simulink model "TASK4"  (R2019a)
settings: Solver=VariableStepAuto  StartTime=0.0  StopTime=30  RelTol=1e-3
values from neighbouring files (symbols this model uses):
  A = [0,mf*g*h/Jconst,0,-(mf*g)/Jconst;1,0,0,0;0,-g,0,0;0,0,1,0]    [Dharmesh_DCS_LAB_Script.m]
  B = [1/Jconst;0;0;0]    [Dharmesh_DCS_LAB_Script.m]
  C = eye(4)    [Dharmesh_DCS_LAB_Script.m]
  D = [0;0;0;0]    [Dharmesh_DCS_LAB_Script.m]
  g = 9.81    [Dharmesh_DCS_LAB_Script.m]
  h = 0.1    [Dharmesh_DCS_LAB_Script.m]
  Jconst = Jb+mf*h^2    (= 0.501)    [Dharmesh_DCS_LAB_Script.m]
  K = q * (alpha(5)*eye(4) + alpha(4)*A + alpha(3)*A^2 + alpha(2)*A^3 + A^4)    [Dharmesh_DCS_LAB_Script.m]
  mf = 0.1    [Dharmesh_DCS_LAB_Script.m]
  P = 1/(Ct*inv((B*K)-A)*B)    [Dharmesh_DCS_LAB_Script.m]
settings Model: Creator=Admin  LastModifiedBy=Admin

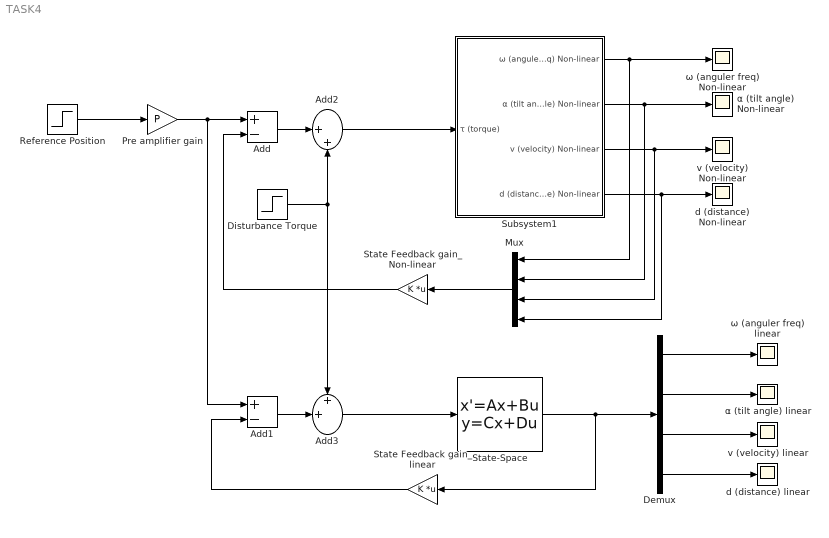
== system TASK4 ==
  "      ω (anguler freq) Non-linear" : Scope
  Add : Sum  Inputs=+-
  Add1 : Sum  Inputs=+-
  Add2 : Sum  Inputs=|++
  Add3 : Sum  Inputs=++|
  Demux : Demux
  Disturbance Torque : Step  Time=15  After=0.1  SampleTime=0
  Mux : Mux
  Pre amplifier gain : Gain  Gain=P
  Reference Position : Step  Time=0  SampleTime=0
  State Feedback gain_Non-linear : Gain  Gain=K  Multiplication=Matrix(K*u) (u vector)
  State Feedback gain_linear : Gain  Gain=K  Multiplication=Matrix(K*u) (u vector)
  State-Space : StateSpace  A=A  B=B  C=C  D=D  InitialCondition=0
  Subsystem1 : Subsystem
  d (distance) Non-linear : Scope
  d (distance) linear : Scope
  v (velocity) Non-linear : Scope
  v (velocity) linear : Scope
  α (tilt angle) Non-linear : Scope
  α (tilt angle) linear : Scope
  ω (anguler freq) linear : Scope
  wires:
  State Feedback gain_Non-linear/1 -> Add/2
  Reference Position/1 -> Pre amplifier gain/1
  State Feedback gain_linear/1 -> Add1/2
  Pre amplifier gain/1 -> Add/1, Add1/1
  Mux/1 -> State Feedback gain_Non-linear/1
  State-Space/1 -> State Feedback gain_linear/1, Demux/1
  Demux/1 -> ω (anguler freq) linear/1
  Demux/2 -> α (tilt angle) linear/1
  Demux/4 -> d (distance) linear/1
  Demux/3 -> v (velocity) linear/1
  Subsystem1/4(d (distance) Non-linear) -> Mux/4, d (distance) Non-linear/1
  Subsystem1/3(v (velocity) Non-linear) -> Mux/3, v (velocity) Non-linear/1
  Subsystem1/2(α (tilt angle) Non-linear) -> Mux/2, α (tilt angle) Non-linear/1
  Subsystem1/1(ω (anguler freq) Non-linear) -> Mux/1, "      ω (anguler freq) Non-linear"/1
  Add2/1 -> Subsystem1/1(τ (torque))
  Add/1 -> Add2/1
  Add1/1 -> Add3/2
  Add3/1 -> State-Space/1
  Disturbance Torque/1 -> Add2/2, Add3/1

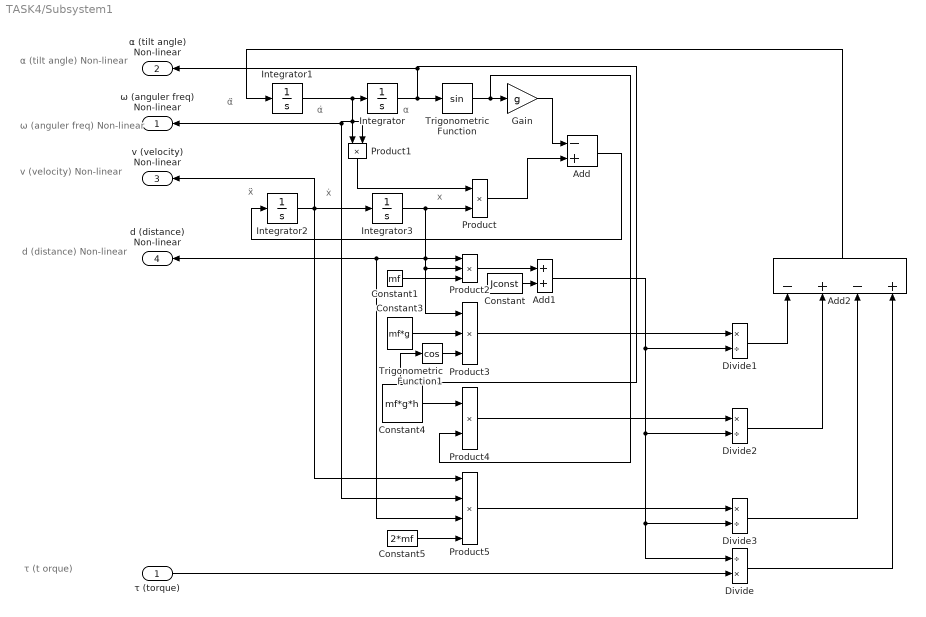
== system TASK4/Subsystem1 ==
  note: α̇
  note: α
  note: ẍ
  note: ẋ
  note: x
  note: τ (t orque)
  note: d (distance) Non-linear
  note: v (velocity) Non-linear
  note: α (tilt angle) Non-linear
  note: ω (anguler freq) Non-linear
  note: α̈
  τ (torque) : Inport
  Add : Sum  Inputs=-+
  Add1 : Sum
  Add2 : Sum  Inputs=-+-+
  Constant : Constant  Value=Jconst
  Constant1 : Constant  Value=mf
  Constant3 : Constant  Value=mf*g
  Constant4 : Constant  Value=mf*g*h
  Constant5 : Constant  Value=2*mf
  Divide : Product  Inputs=/*
  Divide1 : Product  Inputs=*/
  Divide2 : Product  Inputs=*/
  Divide3 : Product  Inputs=*/
  Gain : Gain  Gain=g
  Integrator{,1..3} (4 alike) : Integrator
  Product : Product
  Product1 : Product
  Product2 : Product  Inputs=3
  Product3 : Product  Inputs=3
  Product4 : Product
  Product5 : Product  Inputs=4
  Trigonometric Function : Trigonometry
  Trigonometric Function1 : Trigonometry  Operator=cos
  ω (anguler freq) Non-linear : Outport
  α (tilt angle) Non-linear : Outport  Port=2
  v (velocity) Non-linear : Outport  Port=3
  d (distance) Non-linear : Outport  Port=4
  wires:
  Product2/1 -> Add1/1
  Integrator1/1 -> Product1/2, Product1/1, ω (anguler freq) Non-linear/1, Product5/2, Integrator/1
  Product5/1 -> Divide3/1
  Divide3/1 -> Add2/3
  Product4/1 -> Divide2/1
  Divide/1 -> Add2/4
  Integrator/1 -> Trigonometric Function1/1, α (tilt angle) Non-linear/1, Trigonometric Function/1
  Divide1/1 -> Add2/1
  Product1/1 -> Product/1
  Add1/1 -> Divide/1, Divide3/2, Divide2/2, Divide1/2
  Add/1 -> Integrator2/1
  Trigonometric Function/1 -> Product4/2, Gain/1
  Constant1/1 -> Product2/3
  Product3/1 -> Divide1/1
  Constant3/1 -> Product3/2
  Add2/1 -> Integrator1/1
  Integrator3/1 -> Product/2, Product3/1, Product2/2, d (distance) Non-linear/1, Product5/3, Product2/1
  Divide2/1 -> Add2/2
  Constant4/1 -> Product4/1
  Integrator2/1 -> v (velocity) Non-linear/1, Product5/1, Integrator3/1
  Constant/1 -> Add1/2
  Product/1 -> Add/2
  τ (torque)/1 -> Divide/2
  Constant5/1 -> Product5/4
  Trigonometric Function1/1 -> Product3/3
  Gain/1 -> Add/1
